simulink model "MassSpringMPC_2"  (R2021b)
settings: Solver=FixedStepAuto  StartTime=0.0  StopTime=200  FixedStep=0.1  RelTol=1e-3
PreLoadFcn:
  | load MassSpringMPC_2;
  | load Continuous_Plant_Model;
libraries: mpclib x1, cstblocks x1
settings Model: Creator=wsmur  LastModifiedBy=wsmur

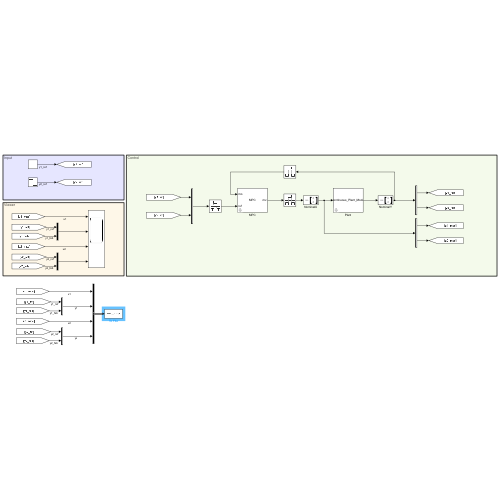
[thumbnail: Simulink's stored preview of the top-level diagram]
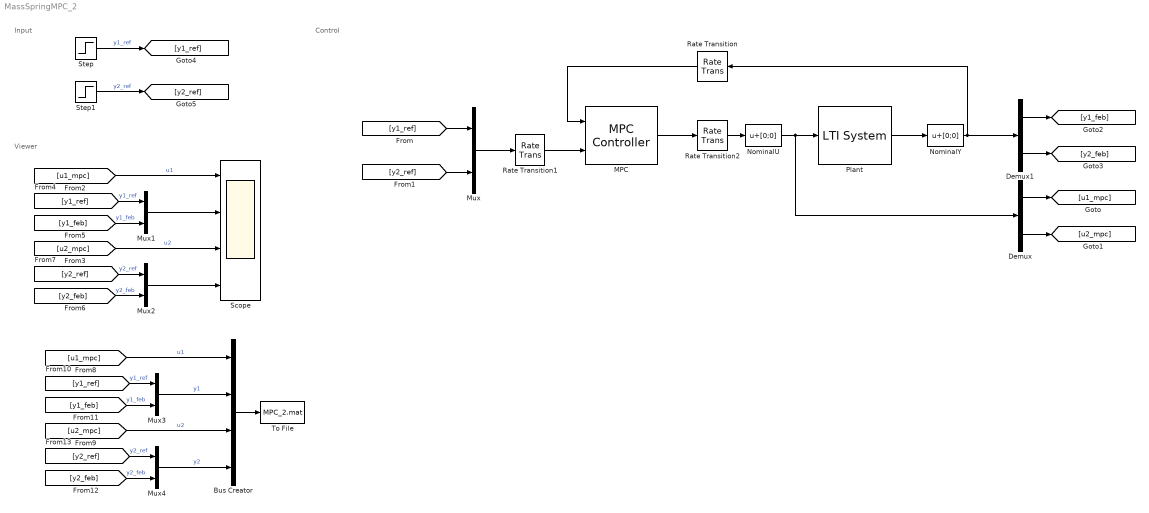
== system MassSpringMPC_2 ==
  note: Control
  note: Input
  note: Viewer
  Bus Creator : BusCreator  Inputs=4
  Demux : Demux  Outputs=2
  Demux1 : Demux  Outputs=2
  MPC : mpclib/MPC Controller  SCDEnableBlockLinearizationSpecification=on  mpcobj=MassSpringMPC_2  is_multiple=0  enable_value=0  return_u0=off  updateMPCinCallerWorkspace=on  md_inport=off  mv_inport=off  uref_inport=off  return_cost=off  return_mvseq=off  return_qpstatus=off  return_xseq=off  return_state=off  return_ovseq=off  state_inport=off  umin_inport=off  umax_inport=off  ymin_inport=off  ymax_inport=off  cc_inport=off  ywt_inport=off  uwt_inport=off  duwt_inport=off  rhoeps_inport=off  pm_inport=off  MaximumP=10  HorizonChoice=FixedHorizon  n_ts=0.1  n_p=10  n_mv=2  n_md=0  n_ud=0  n_mo=2  n_uo=0  BlockDataType=double  SampleTimeInherited=off  switch_inport=off
  Mux{,1..4} (5 alike) : Mux  Inputs=2
  NominalU : Bias  Bias=[0;0]  SaturateOnIntegerOverflow=on
  NominalY : Bias  Bias=[0;0]  SaturateOnIntegerOverflow=on
  Plant : cstblocks/LTI System  sys=Continuous_Plant_Model  IC=[]
  Rate Transition : RateTransition
  Rate Transition1 : RateTransition
  Rate Transition2 : RateTransition
  Scope : Scope  NumInputPorts=4
  Step : Step  Time=50  Before=0.5  After=0.75  SampleTime=0
  Step1 : Step  Time=100  Before=0.6  After=0.3  SampleTime=0
  To File : ToFile  Filename=MPC_2.mat  MatrixName=MPC2  SaveFormat=Timeseries
  wires:
  Mux/1 -> Rate Transition1/1
  Plant/1 -> NominalY/1
  MPC/1 -> Rate Transition2/1
  NominalU/1 -> Demux/1, Plant/1
  Step/1 -> [y1_ref]  "y1_ref"
  Step1/1 -> [y2_ref]  "y2_ref"
  Rate Transition/1 -> MPC/1
  Rate Transition1/1 -> MPC/2
  Rate Transition2/1 -> NominalU/1
  Demux/2 -> [u2_mpc]
  Demux/1 -> [u1_mpc]
  NominalY/1 -> Rate Transition/1, Demux1/1
  Demux1/1 -> [y1_feb]
  Demux1/2 -> [y2_feb]
  [y1_ref] -> Mux/1
  [y2_ref] -> Mux/2
  [y1_ref] -> Mux1/1  "y1_ref"
  [y1_feb] -> Mux1/2  "y1_feb"
  [y2_ref] -> Mux2/1  "y2_ref"
  [y2_feb] -> Mux2/2  "y2_feb"
  Mux1/1 -> Scope/2
  [u1_mpc] -> Scope/1  "u1"
  [u2_mpc] -> Scope/3  "u2"
  Mux2/1 -> Scope/4
  Bus Creator/1 -> To File/1
  [y1_feb] -> Mux3/2  "y1_feb"
  [y2_ref] -> Mux4/1  "y2_ref"
  [u1_mpc] -> Bus Creator/1  "u1"
  Mux3/1 -> Bus Creator/2  "y1"
  [y1_ref] -> Mux3/1  "y1_ref"
  [y2_feb] -> Mux4/2  "y2_feb"
  Mux4/1 -> Bus Creator/4  "y2"
  [u2_mpc] -> Bus Creator/3  "u2"
